simulink library "sandy_sensors"  (R2026a)
settings: Solver=VariableStepAuto
libraries: ros2lib x4

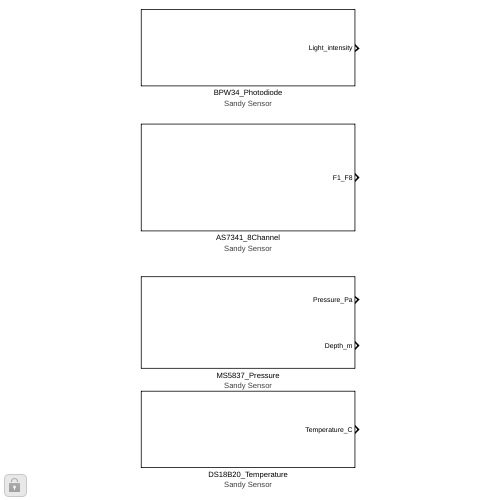
[thumbnail: Simulink's stored preview of the top-level diagram]
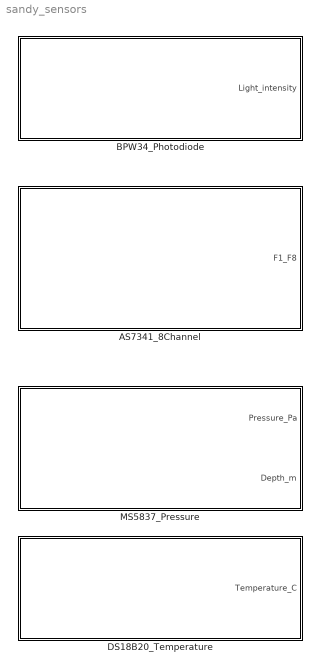
== system sandy_sensors ==
  AS7341_8Channel : Subsystem  Description=AS7341 8-channel proxy. Subscribes to /sandy/as7341_down (sensor_msgs/Image, 8x8 RGB from Gazebo) and synthesises 8 spectral channels F1..F8 (415, 445, 480, 515, 555, 590, 630, 680 nm). Output is uint16(1x8), matching the AS7341 16-bit ADC range. NOTE: This is a synthesis from broadband RGB. Useful for testing detection logic and data pipelines; not physically accurate for spectral retrieval algorithms.
  BPW34_Photodiode : Subsystem  Description=BPW34 photodiode proxy. Subscribes to /sandy/photodiode_side (sensor_msgs/Image, 4x4 RGB from Gazebo) and outputs a scalar irradiance in [0, 1]. Multiply by your photocurrent scale factor (e.g. 5e-7 A) before feeding into the TIA.
  DS18B20_Temperature : Subsystem  Description=DS18B20 temperature proxy. Subscribes to /sandy/temperature (sensor_msgs/Temperature, published by the helper node from the Antarctic depth profile OR a manual slider). Outputs scalar T in C.
  MS5837_Pressure : Subsystem  Description=MS5837-30BA proxy. Subscribes to /sandy/pressure (sensor_msgs/FluidPressure, computed from buoy Z by the helper node). Outputs absolute pressure in Pa AND depth in m (depth = (P - 101325) / (1028 * 9.80665)).

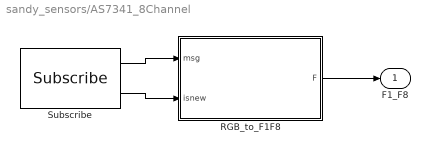
== system sandy_sensors/AS7341_8Channel ==
  RGB_to_F1F8 : MATLAB Function  TreatAsAtomicUnit=on
  Subscribe : ros2lib/Subscribe  topicSource=Specify your own  topic=/sandy/as7341_down  messageType=sensor_msgs/Image  sampleTime=0.1  QOSHistory=Keep last  QOSDepth=5  QOSReliability=Best effort  QOSDurability=Volatile  QOSDeadline=Inf  QOSLifespan=Inf  QOSLiveliness=Automatic  QOSLeaseDuration=Inf  QOSAvoidROSNamespaceConventions=off
  F1_F8 : Outport
  wires:
  Subscribe/1 -> RGB_to_F1F8/1(msg)
  Subscribe/2 -> RGB_to_F1F8/2(isnew)
  RGB_to_F1F8/1(F) -> F1_F8/1

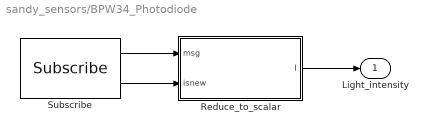
== system sandy_sensors/BPW34_Photodiode ==
  Reduce_to_scalar : MATLAB Function  TreatAsAtomicUnit=on
  Subscribe : ros2lib/Subscribe  topicSource=Specify your own  topic=/sandy/photodiode_side  messageType=sensor_msgs/Image  sampleTime=0.1  QOSHistory=Keep last  QOSDepth=5  QOSReliability=Best effort  QOSDurability=Volatile  QOSDeadline=Inf  QOSLifespan=Inf  QOSLiveliness=Automatic  QOSLeaseDuration=Inf  QOSAvoidROSNamespaceConventions=off
  Light_intensity : Outport
  wires:
  Subscribe/1 -> Reduce_to_scalar/1(msg)
  Subscribe/2 -> Reduce_to_scalar/2(isnew)
  Reduce_to_scalar/1(I) -> Light_intensity/1

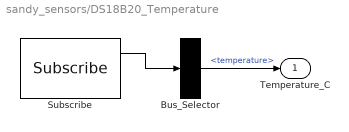
== system sandy_sensors/DS18B20_Temperature ==
  Bus_Selector : BusSelector  OutputSignals=temperature
  Subscribe : ros2lib/Subscribe  topicSource=Specify your own  topic=/sandy/temperature  messageType=sensor_msgs/Temperature  sampleTime=0.1  QOSHistory=Keep last  QOSDepth=5  QOSReliability=Best effort  QOSDurability=Volatile  QOSDeadline=Inf  QOSLifespan=Inf  QOSLiveliness=Automatic  QOSLeaseDuration=Inf  QOSAvoidROSNamespaceConventions=off
  Temperature_C : Outport
  wires:
  Subscribe/1 -> Bus_Selector/1
  Bus_Selector/1 -> Temperature_C/1  "<temperature>"

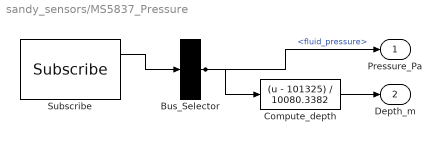
== system sandy_sensors/MS5837_Pressure ==
  Bus_Selector : BusSelector  OutputSignals=fluid_pressure
  Compute_depth : Fcn  Expr=(u - 101325) / 10080.3382
  Subscribe : ros2lib/Subscribe  topicSource=Specify your own  topic=/sandy/pressure  messageType=sensor_msgs/FluidPressure  sampleTime=0.1  QOSHistory=Keep last  QOSDepth=5  QOSReliability=Best effort  QOSDurability=Volatile  QOSDeadline=Inf  QOSLifespan=Inf  QOSLiveliness=Automatic  QOSLeaseDuration=Inf  QOSAvoidROSNamespaceConventions=off
  Pressure_Pa : Outport
  Depth_m : Outport  Port=2
  wires:
  Subscribe/1 -> Bus_Selector/1
  Bus_Selector/1 -> Pressure_Pa/1, Compute_depth/1  "<fluid_pressure>"
  Compute_depth/1 -> Depth_m/1

== matlab function sandy_sensors/BPW34_Photodiode/Reduce_to_scalar ==
function I = reduce(msg, isnew)
%#codegen
% Average all bytes in the image data; normalise to 0..1.
% msg.Data is uint8 array (variable-size).
persistent last_val
if isempty(last_val), last_val = 0; end
if isnew
    n = double(msg.Data_SL_Info.CurrentLength);
    if n > 0
        last_val = double(sum(msg.Data(1:n))) / (n * 255);
    end
end
I = last_val;

== matlab function sandy_sensors/AS7341_8Channel/RGB_to_F1F8 ==
function F = rgb_to_bands(msg, isnew)
%#codegen
% Synthesise 8 AS7341 channels (F1..F8) from a Gazebo RGB image.
% Output F is uint16 1x8, range 0..65535, matching AS7341 ADC.
persistent last
if isempty(last), last = uint16(zeros(1,8)); end
if isnew
    n = double(msg.Data_SL_Info.CurrentLength);
    if mod(n, 3) == 0 && n > 0
        d = double(msg.Data(1:n));
        R = mean(d(1:3:end));
        G = mean(d(2:3:end));
        B = mean(d(3:3:end));
        % 8x3 weight matrix (rows = F1..F8, cols = R G B).
        W = [0.00 0.05 0.95;   % F1 415nm
             0.00 0.10 0.90;   % F2 445nm
             0.00 0.25 0.75;   % F3 480nm
             0.00 0.50 0.50;   % F4 515nm
             0.10 0.80 0.10;   % F5 555nm
             0.30 0.65 0.05;   % F6 590nm
             0.75 0.25 0.00;   % F7 630nm
             0.95 0.05 0.00];  % F8 680nm
        bands = W * [R; G; B];
        % Scale 0..255 (byte) up to 0..65535 (16-bit ADC).
        last = uint16(min(65535, bands * 257));
    end
end
F = last;
